simulink model "simple_router"  (R2015a)
settings: Solver=ode45  StartTime=0.0  StopTime=3000  FixedStep=1  RelTol=1e-3
undefined symbols (not defined in the file or in its folder): des, SELECT, T
libraries: simulink x16
(part 5 of 6)

== system simple_router/Router13/Clocked FIFO5 ==
  Event-Based Random Number : EventBasedRandomNumber  Distribution=Gaussian (normal)  meanNorm=E  stdNorm=S
  FIFO Queue : FIFOQueue  Capacity=F  StatNumberInBlock=on
      settings: OutputPortMap=o1
  Release Gate : ReleaseGate  OpenGateUpon=Function call from port fcn
  Time-Based Function-Call Generator : TimeBasedFunctionCallGenerator  EventGenerationMode=Period from port  Period=T
  Input : PMIOPort  Port=1  Side=Left
  Output : PMIOPort  Port=2  Side=Right
  #n : Outport
  wires:
  Time-Based Function-Call Generator/1 -> Release Gate/1
  FIFO Queue/1 -> #n/1
  Event-Based Random Number/1 -> Time-Based Function-Call Generator/1
  connections:
  FIFO Queue/LConn1 -- Input/RConn1
  Release Gate/RConn1 -- Output/RConn1
  FIFO Queue/RConn1 -- Release Gate/LConn1

== system simple_router/Router20/Attribute Function ==
  MATLAB Function : MATLAB Function  TreatAsAtomicUnit=on
  __DMLF__EDE2FCE__ : EntityDepartureFunctionCallGenerator  TimingFunctionCallF1=Before entity departure  IsInsideAFB=on
  __DMLF__GA__ : GetAttribute  AttributeName=DST|ME  AttributeMissing=Error|Error  AttributeDefaultValue=1|1  AttributeTreatAsVector=1|1  AttributeSendTiming=Before entity departure|Before entity departure  EvaluatedDefaultAttributeValue={ [];[]}  IsInsideAFB=on
      settings: OutputPortMap=o1,o2
  __DMLF__SA__ : SetAttribute  AttributeName=RT  AttributeFrom=Signal port  EvaluatedAttributeValue={ []}  IsInsideAFB=on
  IN : PMIOPort  Port=1  Side=Left
  OUT : PMIOPort  Port=2  Side=Right
  wires:
  __DMLF__EDE2FCE__/1 -> MATLAB Function/Trigger
  __DMLF__GA__/1 -> MATLAB Function/1(DST)
  __DMLF__GA__/2 -> MATLAB Function/2(ME)
  MATLAB Function/1(out_RT) -> __DMLF__SA__/1
  connections:
  __DMLF__SA__/LConn1 -- __DMLF__EDE2FCE__/RConn1
  __DMLF__GA__/RConn1 -- __DMLF__EDE2FCE__/LConn1
  IN/RConn1 -- __DMLF__GA__/LConn1
  __DMLF__SA__/RConn1 -- OUT/RConn1

== system simple_router/Router20/Clocked FIFO1 ==
  Event-Based Random Number : EventBasedRandomNumber  Distribution=Gaussian (normal)  meanNorm=E  stdNorm=S
  FIFO Queue : FIFOQueue  Capacity=F  StatNumberInBlock=on
      settings: OutputPortMap=o1
  Release Gate : ReleaseGate  OpenGateUpon=Function call from port fcn
  Time-Based Function-Call Generator : TimeBasedFunctionCallGenerator  EventGenerationMode=Period from port  Period=T
  Input : PMIOPort  Port=1  Side=Left
  Output : PMIOPort  Port=2  Side=Right
  #n : Outport
  wires:
  Time-Based Function-Call Generator/1 -> Release Gate/1
  FIFO Queue/1 -> #n/1
  Event-Based Random Number/1 -> Time-Based Function-Call Generator/1
  connections:
  FIFO Queue/LConn1 -- Input/RConn1
  Release Gate/RConn1 -- Output/RConn1
  FIFO Queue/RConn1 -- Release Gate/LConn1

== system simple_router/Router20/Clocked FIFO2 ==
  Event-Based Random Number : EventBasedRandomNumber  Distribution=Gaussian (normal)  meanNorm=E  stdNorm=S
  FIFO Queue : FIFOQueue  Capacity=F  StatNumberInBlock=on
      settings: OutputPortMap=o1
  Release Gate : ReleaseGate  OpenGateUpon=Function call from port fcn
  Time-Based Function-Call Generator : TimeBasedFunctionCallGenerator  EventGenerationMode=Period from port  Period=T
  Input : PMIOPort  Port=1  Side=Left
  Output : PMIOPort  Port=2  Side=Right
  #n : Outport
  wires:
  Time-Based Function-Call Generator/1 -> Release Gate/1
  FIFO Queue/1 -> #n/1
  Event-Based Random Number/1 -> Time-Based Function-Call Generator/1
  connections:
  FIFO Queue/LConn1 -- Input/RConn1
  Release Gate/RConn1 -- Output/RConn1
  FIFO Queue/RConn1 -- Release Gate/LConn1

== system simple_router/Router20/Clocked FIFO3 ==
  Event-Based Random Number : EventBasedRandomNumber  Distribution=Gaussian (normal)  meanNorm=E  stdNorm=S
  FIFO Queue : FIFOQueue  Capacity=F  StatNumberInBlock=on
      settings: OutputPortMap=o1
  Release Gate : ReleaseGate  OpenGateUpon=Function call from port fcn
  Time-Based Function-Call Generator : TimeBasedFunctionCallGenerator  EventGenerationMode=Period from port  Period=T
  Input : PMIOPort  Port=1  Side=Left
  Output : PMIOPort  Port=2  Side=Right
  #n : Outport
  wires:
  Time-Based Function-Call Generator/1 -> Release Gate/1
  FIFO Queue/1 -> #n/1
  Event-Based Random Number/1 -> Time-Based Function-Call Generator/1
  connections:
  FIFO Queue/LConn1 -- Input/RConn1
  Release Gate/RConn1 -- Output/RConn1
  FIFO Queue/RConn1 -- Release Gate/LConn1

== system simple_router/Router20/Clocked FIFO4 ==
  Event-Based Random Number : EventBasedRandomNumber  Distribution=Gaussian (normal)  meanNorm=E  stdNorm=S
  FIFO Queue : FIFOQueue  Capacity=F  StatNumberInBlock=on
      settings: OutputPortMap=o1
  Release Gate : ReleaseGate  OpenGateUpon=Function call from port fcn
  Time-Based Function-Call Generator : TimeBasedFunctionCallGenerator  EventGenerationMode=Period from port  Period=T
  Input : PMIOPort  Port=1  Side=Left
  Output : PMIOPort  Port=2  Side=Right
  #n : Outport
  wires:
  Time-Based Function-Call Generator/1 -> Release Gate/1
  FIFO Queue/1 -> #n/1
  Event-Based Random Number/1 -> Time-Based Function-Call Generator/1
  connections:
  FIFO Queue/LConn1 -- Input/RConn1
  Release Gate/RConn1 -- Output/RConn1
  FIFO Queue/RConn1 -- Release Gate/LConn1

== system simple_router/Router20/Clocked FIFO5 ==
  Event-Based Random Number : EventBasedRandomNumber  Distribution=Gaussian (normal)  meanNorm=E  stdNorm=S
  FIFO Queue : FIFOQueue  Capacity=F  StatNumberInBlock=on
      settings: OutputPortMap=o1
  Release Gate : ReleaseGate  OpenGateUpon=Function call from port fcn
  Time-Based Function-Call Generator : TimeBasedFunctionCallGenerator  EventGenerationMode=Period from port  Period=T
  Input : PMIOPort  Port=1  Side=Left
  Output : PMIOPort  Port=2  Side=Right
  #n : Outport
  wires:
  Time-Based Function-Call Generator/1 -> Release Gate/1
  FIFO Queue/1 -> #n/1
  Event-Based Random Number/1 -> Time-Based Function-Call Generator/1
  connections:
  FIFO Queue/LConn1 -- Input/RConn1
  Release Gate/RConn1 -- Output/RConn1
  FIFO Queue/RConn1 -- Release Gate/LConn1

== system simple_router/Router22/Attribute Function ==
  MATLAB Function : MATLAB Function  TreatAsAtomicUnit=on
  __DMLF__EDE2FCE__ : EntityDepartureFunctionCallGenerator  TimingFunctionCallF1=Before entity departure  IsInsideAFB=on
  __DMLF__GA__ : GetAttribute  AttributeName=DST|ME  AttributeMissing=Error|Error  AttributeDefaultValue=1|1  AttributeTreatAsVector=1|1  AttributeSendTiming=Before entity departure|Before entity departure  EvaluatedDefaultAttributeValue={ [];[]}  IsInsideAFB=on
      settings: OutputPortMap=o1,o2
  __DMLF__SA__ : SetAttribute  AttributeName=RT  AttributeFrom=Signal port  EvaluatedAttributeValue={ []}  IsInsideAFB=on
  IN : PMIOPort  Port=1  Side=Left
  OUT : PMIOPort  Port=2  Side=Right
  wires:
  __DMLF__EDE2FCE__/1 -> MATLAB Function/Trigger
  __DMLF__GA__/1 -> MATLAB Function/1(DST)
  __DMLF__GA__/2 -> MATLAB Function/2(ME)
  MATLAB Function/1(out_RT) -> __DMLF__SA__/1
  connections:
  __DMLF__SA__/LConn1 -- __DMLF__EDE2FCE__/RConn1
  __DMLF__GA__/RConn1 -- __DMLF__EDE2FCE__/LConn1
  IN/RConn1 -- __DMLF__GA__/LConn1
  __DMLF__SA__/RConn1 -- OUT/RConn1

== system simple_router/Router22/Clocked FIFO1 ==
  Event-Based Random Number : EventBasedRandomNumber  Distribution=Gaussian (normal)  meanNorm=E  stdNorm=S
  FIFO Queue : FIFOQueue  Capacity=F  StatNumberInBlock=on
      settings: OutputPortMap=o1
  Release Gate : ReleaseGate  OpenGateUpon=Function call from port fcn
  Time-Based Function-Call Generator : TimeBasedFunctionCallGenerator  EventGenerationMode=Period from port  Period=T
  Input : PMIOPort  Port=1  Side=Left
  Output : PMIOPort  Port=2  Side=Right
  #n : Outport
  wires:
  Time-Based Function-Call Generator/1 -> Release Gate/1
  FIFO Queue/1 -> #n/1
  Event-Based Random Number/1 -> Time-Based Function-Call Generator/1
  connections:
  FIFO Queue/LConn1 -- Input/RConn1
  Release Gate/RConn1 -- Output/RConn1
  FIFO Queue/RConn1 -- Release Gate/LConn1

== system simple_router/Router22/Clocked FIFO2 ==
  Event-Based Random Number : EventBasedRandomNumber  Distribution=Gaussian (normal)  meanNorm=E  stdNorm=S
  FIFO Queue : FIFOQueue  Capacity=F  StatNumberInBlock=on
      settings: OutputPortMap=o1
  Release Gate : ReleaseGate  OpenGateUpon=Function call from port fcn
  Time-Based Function-Call Generator : TimeBasedFunctionCallGenerator  EventGenerationMode=Period from port  Period=T
  Input : PMIOPort  Port=1  Side=Left
  Output : PMIOPort  Port=2  Side=Right
  #n : Outport
  wires:
  Time-Based Function-Call Generator/1 -> Release Gate/1
  FIFO Queue/1 -> #n/1
  Event-Based Random Number/1 -> Time-Based Function-Call Generator/1
  connections:
  FIFO Queue/LConn1 -- Input/RConn1
  Release Gate/RConn1 -- Output/RConn1
  FIFO Queue/RConn1 -- Release Gate/LConn1

== system simple_router/Router22/Clocked FIFO3 ==
  Event-Based Random Number : EventBasedRandomNumber  Distribution=Gaussian (normal)  meanNorm=E  stdNorm=S
  FIFO Queue : FIFOQueue  Capacity=F  StatNumberInBlock=on
      settings: OutputPortMap=o1
  Release Gate : ReleaseGate  OpenGateUpon=Function call from port fcn
  Time-Based Function-Call Generator : TimeBasedFunctionCallGenerator  EventGenerationMode=Period from port  Period=T
  Input : PMIOPort  Port=1  Side=Left
  Output : PMIOPort  Port=2  Side=Right
  #n : Outport
  wires:
  Time-Based Function-Call Generator/1 -> Release Gate/1
  FIFO Queue/1 -> #n/1
  Event-Based Random Number/1 -> Time-Based Function-Call Generator/1
  connections:
  FIFO Queue/LConn1 -- Input/RConn1
  Release Gate/RConn1 -- Output/RConn1
  FIFO Queue/RConn1 -- Release Gate/LConn1

== system simple_router/Router22/Clocked FIFO4 ==
  Event-Based Random Number : EventBasedRandomNumber  Distribution=Gaussian (normal)  meanNorm=E  stdNorm=S
  FIFO Queue : FIFOQueue  Capacity=F  StatNumberInBlock=on
      settings: OutputPortMap=o1
  Release Gate : ReleaseGate  OpenGateUpon=Function call from port fcn
  Time-Based Function-Call Generator : TimeBasedFunctionCallGenerator  EventGenerationMode=Period from port  Period=T
  Input : PMIOPort  Port=1  Side=Left
  Output : PMIOPort  Port=2  Side=Right
  #n : Outport
  wires:
  Time-Based Function-Call Generator/1 -> Release Gate/1
  FIFO Queue/1 -> #n/1
  Event-Based Random Number/1 -> Time-Based Function-Call Generator/1
  connections:
  FIFO Queue/LConn1 -- Input/RConn1
  Release Gate/RConn1 -- Output/RConn1
  FIFO Queue/RConn1 -- Release Gate/LConn1

== system simple_router/Router22/Clocked FIFO5 ==
  Event-Based Random Number : EventBasedRandomNumber  Distribution=Gaussian (normal)  meanNorm=E  stdNorm=S
  FIFO Queue : FIFOQueue  Capacity=F  StatNumberInBlock=on
      settings: OutputPortMap=o1
  Release Gate : ReleaseGate  OpenGateUpon=Function call from port fcn
  Time-Based Function-Call Generator : TimeBasedFunctionCallGenerator  EventGenerationMode=Period from port  Period=T
  Input : PMIOPort  Port=1  Side=Left
  Output : PMIOPort  Port=2  Side=Right
  #n : Outport
  wires:
  Time-Based Function-Call Generator/1 -> Release Gate/1
  FIFO Queue/1 -> #n/1
  Event-Based Random Number/1 -> Time-Based Function-Call Generator/1
  connections:
  FIFO Queue/LConn1 -- Input/RConn1
  Release Gate/RConn1 -- Output/RConn1
  FIFO Queue/RConn1 -- Release Gate/LConn1

== system simple_router/Router23/Attribute Function ==
  MATLAB Function : MATLAB Function  TreatAsAtomicUnit=on
  __DMLF__EDE2FCE__ : EntityDepartureFunctionCallGenerator  TimingFunctionCallF1=Before entity departure  IsInsideAFB=on
  __DMLF__GA__ : GetAttribute  AttributeName=DST|ME  AttributeMissing=Error|Error  AttributeDefaultValue=1|1  AttributeTreatAsVector=1|1  AttributeSendTiming=Before entity departure|Before entity departure  EvaluatedDefaultAttributeValue={ [];[]}  IsInsideAFB=on
      settings: OutputPortMap=o1,o2
  __DMLF__SA__ : SetAttribute  AttributeName=RT  AttributeFrom=Signal port  EvaluatedAttributeValue={ []}  IsInsideAFB=on
  IN : PMIOPort  Port=1  Side=Left
  OUT : PMIOPort  Port=2  Side=Right
  wires:
  __DMLF__EDE2FCE__/1 -> MATLAB Function/Trigger
  __DMLF__GA__/1 -> MATLAB Function/1(DST)
  __DMLF__GA__/2 -> MATLAB Function/2(ME)
  MATLAB Function/1(out_RT) -> __DMLF__SA__/1
  connections:
  __DMLF__SA__/LConn1 -- __DMLF__EDE2FCE__/RConn1
  __DMLF__GA__/RConn1 -- __DMLF__EDE2FCE__/LConn1
  IN/RConn1 -- __DMLF__GA__/LConn1
  __DMLF__SA__/RConn1 -- OUT/RConn1

== system simple_router/Router23/Clocked FIFO1 ==
  Event-Based Random Number : EventBasedRandomNumber  Distribution=Gaussian (normal)  meanNorm=E  stdNorm=S
  FIFO Queue : FIFOQueue  Capacity=F  StatNumberInBlock=on
      settings: OutputPortMap=o1
  Release Gate : ReleaseGate  OpenGateUpon=Function call from port fcn
  Time-Based Function-Call Generator : TimeBasedFunctionCallGenerator  EventGenerationMode=Period from port  Period=T
  Input : PMIOPort  Port=1  Side=Left
  Output : PMIOPort  Port=2  Side=Right
  #n : Outport
  wires:
  Time-Based Function-Call Generator/1 -> Release Gate/1
  FIFO Queue/1 -> #n/1
  Event-Based Random Number/1 -> Time-Based Function-Call Generator/1
  connections:
  FIFO Queue/LConn1 -- Input/RConn1
  Release Gate/RConn1 -- Output/RConn1
  FIFO Queue/RConn1 -- Release Gate/LConn1

== system simple_router/Router23/Clocked FIFO2 ==
  Event-Based Random Number : EventBasedRandomNumber  Distribution=Gaussian (normal)  meanNorm=E  stdNorm=S
  FIFO Queue : FIFOQueue  Capacity=F  StatNumberInBlock=on
      settings: OutputPortMap=o1
  Release Gate : ReleaseGate  OpenGateUpon=Function call from port fcn
  Time-Based Function-Call Generator : TimeBasedFunctionCallGenerator  EventGenerationMode=Period from port  Period=T
  Input : PMIOPort  Port=1  Side=Left
  Output : PMIOPort  Port=2  Side=Right
  #n : Outport
  wires:
  Time-Based Function-Call Generator/1 -> Release Gate/1
  FIFO Queue/1 -> #n/1
  Event-Based Random Number/1 -> Time-Based Function-Call Generator/1
  connections:
  FIFO Queue/LConn1 -- Input/RConn1
  Release Gate/RConn1 -- Output/RConn1
  FIFO Queue/RConn1 -- Release Gate/LConn1

== system simple_router/Router23/Clocked FIFO3 ==
  Event-Based Random Number : EventBasedRandomNumber  Distribution=Gaussian (normal)  meanNorm=E  stdNorm=S
  FIFO Queue : FIFOQueue  Capacity=F  StatNumberInBlock=on
      settings: OutputPortMap=o1
  Release Gate : ReleaseGate  OpenGateUpon=Function call from port fcn
  Time-Based Function-Call Generator : TimeBasedFunctionCallGenerator  EventGenerationMode=Period from port  Period=T
  Input : PMIOPort  Port=1  Side=Left
  Output : PMIOPort  Port=2  Side=Right
  #n : Outport
  wires:
  Time-Based Function-Call Generator/1 -> Release Gate/1
  FIFO Queue/1 -> #n/1
  Event-Based Random Number/1 -> Time-Based Function-Call Generator/1
  connections:
  FIFO Queue/LConn1 -- Input/RConn1
  Release Gate/RConn1 -- Output/RConn1
  FIFO Queue/RConn1 -- Release Gate/LConn1

== system simple_router/Router23/Clocked FIFO4 ==
  Event-Based Random Number : EventBasedRandomNumber  Distribution=Gaussian (normal)  meanNorm=E  stdNorm=S
  FIFO Queue : FIFOQueue  Capacity=F  StatNumberInBlock=on
      settings: OutputPortMap=o1
  Release Gate : ReleaseGate  OpenGateUpon=Function call from port fcn
  Time-Based Function-Call Generator : TimeBasedFunctionCallGenerator  EventGenerationMode=Period from port  Period=T
  Input : PMIOPort  Port=1  Side=Left
  Output : PMIOPort  Port=2  Side=Right
  #n : Outport
  wires:
  Time-Based Function-Call Generator/1 -> Release Gate/1
  FIFO Queue/1 -> #n/1
  Event-Based Random Number/1 -> Time-Based Function-Call Generator/1
  connections:
  FIFO Queue/LConn1 -- Input/RConn1
  Release Gate/RConn1 -- Output/RConn1
  FIFO Queue/RConn1 -- Release Gate/LConn1

== system simple_router/Router23/Clocked FIFO5 ==
  Event-Based Random Number : EventBasedRandomNumber  Distribution=Gaussian (normal)  meanNorm=E  stdNorm=S
  FIFO Queue : FIFOQueue  Capacity=F  StatNumberInBlock=on
      settings: OutputPortMap=o1
  Release Gate : ReleaseGate  OpenGateUpon=Function call from port fcn
  Time-Based Function-Call Generator : TimeBasedFunctionCallGenerator  EventGenerationMode=Period from port  Period=T
  Input : PMIOPort  Port=1  Side=Left
  Output : PMIOPort  Port=2  Side=Right
  #n : Outport
  wires:
  Time-Based Function-Call Generator/1 -> Release Gate/1
  FIFO Queue/1 -> #n/1
  Event-Based Random Number/1 -> Time-Based Function-Call Generator/1
  connections:
  FIFO Queue/LConn1 -- Input/RConn1
  Release Gate/RConn1 -- Output/RConn1
  FIFO Queue/RConn1 -- Release Gate/LConn1

== system simple_router/Router30/Attribute Function ==
  MATLAB Function : MATLAB Function  TreatAsAtomicUnit=on
  __DMLF__EDE2FCE__ : EntityDepartureFunctionCallGenerator  TimingFunctionCallF1=Before entity departure  IsInsideAFB=on
  __DMLF__GA__ : GetAttribute  AttributeName=DST|ME  AttributeMissing=Error|Error  AttributeDefaultValue=1|1  AttributeTreatAsVector=1|1  AttributeSendTiming=Before entity departure|Before entity departure  EvaluatedDefaultAttributeValue={ [];[]}  IsInsideAFB=on
      settings: OutputPortMap=o1,o2
  __DMLF__SA__ : SetAttribute  AttributeName=RT  AttributeFrom=Signal port  EvaluatedAttributeValue={ []}  IsInsideAFB=on
  IN : PMIOPort  Port=1  Side=Left
  OUT : PMIOPort  Port=2  Side=Right
  wires:
  __DMLF__EDE2FCE__/1 -> MATLAB Function/Trigger
  __DMLF__GA__/1 -> MATLAB Function/1(DST)
  __DMLF__GA__/2 -> MATLAB Function/2(ME)
  MATLAB Function/1(out_RT) -> __DMLF__SA__/1
  connections:
  __DMLF__SA__/LConn1 -- __DMLF__EDE2FCE__/RConn1
  __DMLF__GA__/RConn1 -- __DMLF__EDE2FCE__/LConn1
  IN/RConn1 -- __DMLF__GA__/LConn1
  __DMLF__SA__/RConn1 -- OUT/RConn1

== system simple_router/Router30/Clocked FIFO1 ==
  Event-Based Random Number : EventBasedRandomNumber  Distribution=Gaussian (normal)  meanNorm=E  stdNorm=S
  FIFO Queue : FIFOQueue  Capacity=F  StatNumberInBlock=on
      settings: OutputPortMap=o1
  Release Gate : ReleaseGate  OpenGateUpon=Function call from port fcn
  Time-Based Function-Call Generator : TimeBasedFunctionCallGenerator  EventGenerationMode=Period from port  Period=T
  Input : PMIOPort  Port=1  Side=Left
  Output : PMIOPort  Port=2  Side=Right
  #n : Outport
  wires:
  Time-Based Function-Call Generator/1 -> Release Gate/1
  FIFO Queue/1 -> #n/1
  Event-Based Random Number/1 -> Time-Based Function-Call Generator/1
  connections:
  FIFO Queue/LConn1 -- Input/RConn1
  Release Gate/RConn1 -- Output/RConn1
  FIFO Queue/RConn1 -- Release Gate/LConn1

== system simple_router/Router30/Clocked FIFO2 ==
  Event-Based Random Number : EventBasedRandomNumber  Distribution=Gaussian (normal)  meanNorm=E  stdNorm=S
  FIFO Queue : FIFOQueue  Capacity=F  StatNumberInBlock=on
      settings: OutputPortMap=o1
  Release Gate : ReleaseGate  OpenGateUpon=Function call from port fcn
  Time-Based Function-Call Generator : TimeBasedFunctionCallGenerator  EventGenerationMode=Period from port  Period=T
  Input : PMIOPort  Port=1  Side=Left
  Output : PMIOPort  Port=2  Side=Right
  #n : Outport
  wires:
  Time-Based Function-Call Generator/1 -> Release Gate/1
  FIFO Queue/1 -> #n/1
  Event-Based Random Number/1 -> Time-Based Function-Call Generator/1
  connections:
  FIFO Queue/LConn1 -- Input/RConn1
  Release Gate/RConn1 -- Output/RConn1
  FIFO Queue/RConn1 -- Release Gate/LConn1

== system simple_router/Router30/Clocked FIFO3 ==
  Event-Based Random Number : EventBasedRandomNumber  Distribution=Gaussian (normal)  meanNorm=E  stdNorm=S
  FIFO Queue : FIFOQueue  Capacity=F  StatNumberInBlock=on
      settings: OutputPortMap=o1
  Release Gate : ReleaseGate  OpenGateUpon=Function call from port fcn
  Time-Based Function-Call Generator : TimeBasedFunctionCallGenerator  EventGenerationMode=Period from port  Period=T
  Input : PMIOPort  Port=1  Side=Left
  Output : PMIOPort  Port=2  Side=Right
  #n : Outport
  wires:
  Time-Based Function-Call Generator/1 -> Release Gate/1
  FIFO Queue/1 -> #n/1
  Event-Based Random Number/1 -> Time-Based Function-Call Generator/1
  connections:
  FIFO Queue/LConn1 -- Input/RConn1
  Release Gate/RConn1 -- Output/RConn1
  FIFO Queue/RConn1 -- Release Gate/LConn1

== system simple_router/Router30/Clocked FIFO4 ==
  Event-Based Random Number : EventBasedRandomNumber  Distribution=Gaussian (normal)  meanNorm=E  stdNorm=S
  FIFO Queue : FIFOQueue  Capacity=F  StatNumberInBlock=on
      settings: OutputPortMap=o1
  Release Gate : ReleaseGate  OpenGateUpon=Function call from port fcn
  Time-Based Function-Call Generator : TimeBasedFunctionCallGenerator  EventGenerationMode=Period from port  Period=T
  Input : PMIOPort  Port=1  Side=Left
  Output : PMIOPort  Port=2  Side=Right
  #n : Outport
  wires:
  Time-Based Function-Call Generator/1 -> Release Gate/1
  FIFO Queue/1 -> #n/1
  Event-Based Random Number/1 -> Time-Based Function-Call Generator/1
  connections:
  FIFO Queue/LConn1 -- Input/RConn1
  Release Gate/RConn1 -- Output/RConn1
  FIFO Queue/RConn1 -- Release Gate/LConn1

== system simple_router/Router30/Clocked FIFO5 ==
  Event-Based Random Number : EventBasedRandomNumber  Distribution=Gaussian (normal)  meanNorm=E  stdNorm=S
  FIFO Queue : FIFOQueue  Capacity=F  StatNumberInBlock=on
      settings: OutputPortMap=o1
  Release Gate : ReleaseGate  OpenGateUpon=Function call from port fcn
  Time-Based Function-Call Generator : TimeBasedFunctionCallGenerator  EventGenerationMode=Period from port  Period=T
  Input : PMIOPort  Port=1  Side=Left
  Output : PMIOPort  Port=2  Side=Right
  #n : Outport
  wires:
  Time-Based Function-Call Generator/1 -> Release Gate/1
  FIFO Queue/1 -> #n/1
  Event-Based Random Number/1 -> Time-Based Function-Call Generator/1
  connections:
  FIFO Queue/LConn1 -- Input/RConn1
  Release Gate/RConn1 -- Output/RConn1
  FIFO Queue/RConn1 -- Release Gate/LConn1

== system simple_router/Router31/Attribute Function ==
  MATLAB Function : MATLAB Function  TreatAsAtomicUnit=on
  __DMLF__EDE2FCE__ : EntityDepartureFunctionCallGenerator  TimingFunctionCallF1=Before entity departure  IsInsideAFB=on
  __DMLF__GA__ : GetAttribute  AttributeName=DST|ME  AttributeMissing=Error|Error  AttributeDefaultValue=1|1  AttributeTreatAsVector=1|1  AttributeSendTiming=Before entity departure|Before entity departure  EvaluatedDefaultAttributeValue={ [];[]}  IsInsideAFB=on
      settings: OutputPortMap=o1,o2
  __DMLF__SA__ : SetAttribute  AttributeName=RT  AttributeFrom=Signal port  EvaluatedAttributeValue={ []}  IsInsideAFB=on
  IN : PMIOPort  Port=1  Side=Left
  OUT : PMIOPort  Port=2  Side=Right
  wires:
  __DMLF__EDE2FCE__/1 -> MATLAB Function/Trigger
  __DMLF__GA__/1 -> MATLAB Function/1(DST)
  __DMLF__GA__/2 -> MATLAB Function/2(ME)
  MATLAB Function/1(out_RT) -> __DMLF__SA__/1
  connections:
  __DMLF__SA__/LConn1 -- __DMLF__EDE2FCE__/RConn1
  __DMLF__GA__/RConn1 -- __DMLF__EDE2FCE__/LConn1
  IN/RConn1 -- __DMLF__GA__/LConn1
  __DMLF__SA__/RConn1 -- OUT/RConn1

== system simple_router/Router31/Clocked FIFO1 ==
  Event-Based Random Number : EventBasedRandomNumber  Distribution=Gaussian (normal)  meanNorm=E  stdNorm=S
  FIFO Queue : FIFOQueue  Capacity=F  StatNumberInBlock=on
      settings: OutputPortMap=o1
  Release Gate : ReleaseGate  OpenGateUpon=Function call from port fcn
  Time-Based Function-Call Generator : TimeBasedFunctionCallGenerator  EventGenerationMode=Period from port  Period=T
  Input : PMIOPort  Port=1  Side=Left
  Output : PMIOPort  Port=2  Side=Right
  #n : Outport
  wires:
  Time-Based Function-Call Generator/1 -> Release Gate/1
  FIFO Queue/1 -> #n/1
  Event-Based Random Number/1 -> Time-Based Function-Call Generator/1
  connections:
  FIFO Queue/LConn1 -- Input/RConn1
  Release Gate/RConn1 -- Output/RConn1
  FIFO Queue/RConn1 -- Release Gate/LConn1

== system simple_router/Router31/Clocked FIFO2 ==
  Event-Based Random Number : EventBasedRandomNumber  Distribution=Gaussian (normal)  meanNorm=E  stdNorm=S
  FIFO Queue : FIFOQueue  Capacity=F  StatNumberInBlock=on
      settings: OutputPortMap=o1
  Release Gate : ReleaseGate  OpenGateUpon=Function call from port fcn
  Time-Based Function-Call Generator : TimeBasedFunctionCallGenerator  EventGenerationMode=Period from port  Period=T
  Input : PMIOPort  Port=1  Side=Left
  Output : PMIOPort  Port=2  Side=Right
  #n : Outport
  wires:
  Time-Based Function-Call Generator/1 -> Release Gate/1
  FIFO Queue/1 -> #n/1
  Event-Based Random Number/1 -> Time-Based Function-Call Generator/1
  connections:
  FIFO Queue/LConn1 -- Input/RConn1
  Release Gate/RConn1 -- Output/RConn1
  FIFO Queue/RConn1 -- Release Gate/LConn1

== system simple_router/Router31/Clocked FIFO3 ==
  Event-Based Random Number : EventBasedRandomNumber  Distribution=Gaussian (normal)  meanNorm=E  stdNorm=S
  FIFO Queue : FIFOQueue  Capacity=F  StatNumberInBlock=on
      settings: OutputPortMap=o1
  Release Gate : ReleaseGate  OpenGateUpon=Function call from port fcn
  Time-Based Function-Call Generator : TimeBasedFunctionCallGenerator  EventGenerationMode=Period from port  Period=T
  Input : PMIOPort  Port=1  Side=Left
  Output : PMIOPort  Port=2  Side=Right
  #n : Outport
  wires:
  Time-Based Function-Call Generator/1 -> Release Gate/1
  FIFO Queue/1 -> #n/1
  Event-Based Random Number/1 -> Time-Based Function-Call Generator/1
  connections:
  FIFO Queue/LConn1 -- Input/RConn1
  Release Gate/RConn1 -- Output/RConn1
  FIFO Queue/RConn1 -- Release Gate/LConn1

== system simple_router/Router31/Clocked FIFO4 ==
  Event-Based Random Number : EventBasedRandomNumber  Distribution=Gaussian (normal)  meanNorm=E  stdNorm=S
  FIFO Queue : FIFOQueue  Capacity=F  StatNumberInBlock=on
      settings: OutputPortMap=o1
  Release Gate : ReleaseGate  OpenGateUpon=Function call from port fcn
  Time-Based Function-Call Generator : TimeBasedFunctionCallGenerator  EventGenerationMode=Period from port  Period=T
  Input : PMIOPort  Port=1  Side=Left
  Output : PMIOPort  Port=2  Side=Right
  #n : Outport
  wires:
  Time-Based Function-Call Generator/1 -> Release Gate/1
  FIFO Queue/1 -> #n/1
  Event-Based Random Number/1 -> Time-Based Function-Call Generator/1
  connections:
  FIFO Queue/LConn1 -- Input/RConn1
  Release Gate/RConn1 -- Output/RConn1
  FIFO Queue/RConn1 -- Release Gate/LConn1

== system simple_router/Router31/Clocked FIFO5 ==
  Event-Based Random Number : EventBasedRandomNumber  Distribution=Gaussian (normal)  meanNorm=E  stdNorm=S
  FIFO Queue : FIFOQueue  Capacity=F  StatNumberInBlock=on
      settings: OutputPortMap=o1
  Release Gate : ReleaseGate  OpenGateUpon=Function call from port fcn
  Time-Based Function-Call Generator : TimeBasedFunctionCallGenerator  EventGenerationMode=Period from port  Period=T
  Input : PMIOPort  Port=1  Side=Left
  Output : PMIOPort  Port=2  Side=Right
  #n : Outport
  wires:
  Time-Based Function-Call Generator/1 -> Release Gate/1
  FIFO Queue/1 -> #n/1
  Event-Based Random Number/1 -> Time-Based Function-Call Generator/1
  connections:
  FIFO Queue/LConn1 -- Input/RConn1
  Release Gate/RConn1 -- Output/RConn1
  FIFO Queue/RConn1 -- Release Gate/LConn1

== system simple_router/Router32/Attribute Function ==
  MATLAB Function : MATLAB Function  TreatAsAtomicUnit=on
  __DMLF__EDE2FCE__ : EntityDepartureFunctionCallGenerator  TimingFunctionCallF1=Before entity departure  IsInsideAFB=on
  __DMLF__GA__ : GetAttribute  AttributeName=DST|ME  AttributeMissing=Error|Error  AttributeDefaultValue=1|1  AttributeTreatAsVector=1|1  AttributeSendTiming=Before entity departure|Before entity departure  EvaluatedDefaultAttributeValue={ [];[]}  IsInsideAFB=on
      settings: OutputPortMap=o1,o2
  __DMLF__SA__ : SetAttribute  AttributeName=RT  AttributeFrom=Signal port  EvaluatedAttributeValue={ []}  IsInsideAFB=on
  IN : PMIOPort  Port=1  Side=Left
  OUT : PMIOPort  Port=2  Side=Right
  wires:
  __DMLF__EDE2FCE__/1 -> MATLAB Function/Trigger
  __DMLF__GA__/1 -> MATLAB Function/1(DST)
  __DMLF__GA__/2 -> MATLAB Function/2(ME)
  MATLAB Function/1(out_RT) -> __DMLF__SA__/1
  connections:
  __DMLF__SA__/LConn1 -- __DMLF__EDE2FCE__/RConn1
  __DMLF__GA__/RConn1 -- __DMLF__EDE2FCE__/LConn1
  IN/RConn1 -- __DMLF__GA__/LConn1
  __DMLF__SA__/RConn1 -- OUT/RConn1

== system simple_router/Router32/Clocked FIFO1 ==
  Event-Based Random Number : EventBasedRandomNumber  Distribution=Gaussian (normal)  meanNorm=E  stdNorm=S
  FIFO Queue : FIFOQueue  Capacity=F  StatNumberInBlock=on
      settings: OutputPortMap=o1
  Release Gate : ReleaseGate  OpenGateUpon=Function call from port fcn
  Time-Based Function-Call Generator : TimeBasedFunctionCallGenerator  EventGenerationMode=Period from port  Period=T
  Input : PMIOPort  Port=1  Side=Left
  Output : PMIOPort  Port=2  Side=Right
  #n : Outport
  wires:
  Time-Based Function-Call Generator/1 -> Release Gate/1
  FIFO Queue/1 -> #n/1
  Event-Based Random Number/1 -> Time-Based Function-Call Generator/1
  connections:
  FIFO Queue/LConn1 -- Input/RConn1
  Release Gate/RConn1 -- Output/RConn1
  FIFO Queue/RConn1 -- Release Gate/LConn1

== system simple_router/Router32/Clocked FIFO2 ==
  Event-Based Random Number : EventBasedRandomNumber  Distribution=Gaussian (normal)  meanNorm=E  stdNorm=S
  FIFO Queue : FIFOQueue  Capacity=F  StatNumberInBlock=on
      settings: OutputPortMap=o1
  Release Gate : ReleaseGate  OpenGateUpon=Function call from port fcn
  Time-Based Function-Call Generator : TimeBasedFunctionCallGenerator  EventGenerationMode=Period from port  Period=T
  Input : PMIOPort  Port=1  Side=Left
  Output : PMIOPort  Port=2  Side=Right
  #n : Outport
  wires:
  Time-Based Function-Call Generator/1 -> Release Gate/1
  FIFO Queue/1 -> #n/1
  Event-Based Random Number/1 -> Time-Based Function-Call Generator/1
  connections:
  FIFO Queue/LConn1 -- Input/RConn1
  Release Gate/RConn1 -- Output/RConn1
  FIFO Queue/RConn1 -- Release Gate/LConn1

== system simple_router/Router32/Clocked FIFO3 ==
  Event-Based Random Number : EventBasedRandomNumber  Distribution=Gaussian (normal)  meanNorm=E  stdNorm=S
  FIFO Queue : FIFOQueue  Capacity=F  StatNumberInBlock=on
      settings: OutputPortMap=o1
  Release Gate : ReleaseGate  OpenGateUpon=Function call from port fcn
  Time-Based Function-Call Generator : TimeBasedFunctionCallGenerator  EventGenerationMode=Period from port  Period=T
  Input : PMIOPort  Port=1  Side=Left
  Output : PMIOPort  Port=2  Side=Right
  #n : Outport
  wires:
  Time-Based Function-Call Generator/1 -> Release Gate/1
  FIFO Queue/1 -> #n/1
  Event-Based Random Number/1 -> Time-Based Function-Call Generator/1
  connections:
  FIFO Queue/LConn1 -- Input/RConn1
  Release Gate/RConn1 -- Output/RConn1
  FIFO Queue/RConn1 -- Release Gate/LConn1

== system simple_router/Router32/Clocked FIFO4 ==
  Event-Based Random Number : EventBasedRandomNumber  Distribution=Gaussian (normal)  meanNorm=E  stdNorm=S
  FIFO Queue : FIFOQueue  Capacity=F  StatNumberInBlock=on
      settings: OutputPortMap=o1
  Release Gate : ReleaseGate  OpenGateUpon=Function call from port fcn
  Time-Based Function-Call Generator : TimeBasedFunctionCallGenerator  EventGenerationMode=Period from port  Period=T
  Input : PMIOPort  Port=1  Side=Left
  Output : PMIOPort  Port=2  Side=Right
  #n : Outport
  wires:
  Time-Based Function-Call Generator/1 -> Release Gate/1
  FIFO Queue/1 -> #n/1
  Event-Based Random Number/1 -> Time-Based Function-Call Generator/1
  connections:
  FIFO Queue/LConn1 -- Input/RConn1
  Release Gate/RConn1 -- Output/RConn1
  FIFO Queue/RConn1 -- Release Gate/LConn1

== system simple_router/Router32/Clocked FIFO5 ==
  Event-Based Random Number : EventBasedRandomNumber  Distribution=Gaussian (normal)  meanNorm=E  stdNorm=S
  FIFO Queue : FIFOQueue  Capacity=F  StatNumberInBlock=on
      settings: OutputPortMap=o1
  Release Gate : ReleaseGate  OpenGateUpon=Function call from port fcn
  Time-Based Function-Call Generator : TimeBasedFunctionCallGenerator  EventGenerationMode=Period from port  Period=T
  Input : PMIOPort  Port=1  Side=Left
  Output : PMIOPort  Port=2  Side=Right
  #n : Outport
  wires:
  Time-Based Function-Call Generator/1 -> Release Gate/1
  FIFO Queue/1 -> #n/1
  Event-Based Random Number/1 -> Time-Based Function-Call Generator/1
  connections:
  FIFO Queue/LConn1 -- Input/RConn1
  Release Gate/RConn1 -- Output/RConn1
  FIFO Queue/RConn1 -- Release Gate/LConn1

== system simple_router/Router33/Attribute Function ==
  MATLAB Function : MATLAB Function  TreatAsAtomicUnit=on
  __DMLF__EDE2FCE__ : EntityDepartureFunctionCallGenerator  TimingFunctionCallF1=Before entity departure  IsInsideAFB=on
  __DMLF__GA__ : GetAttribute  AttributeName=DST|ME  AttributeMissing=Error|Error  AttributeDefaultValue=1|1  AttributeTreatAsVector=1|1  AttributeSendTiming=Before entity departure|Before entity departure  EvaluatedDefaultAttributeValue={ [];[]}  IsInsideAFB=on
      settings: OutputPortMap=o1,o2
  __DMLF__SA__ : SetAttribute  AttributeName=RT  AttributeFrom=Signal port  EvaluatedAttributeValue={ []}  IsInsideAFB=on
  IN : PMIOPort  Port=1  Side=Left
  OUT : PMIOPort  Port=2  Side=Right
  wires:
  __DMLF__EDE2FCE__/1 -> MATLAB Function/Trigger
  __DMLF__GA__/1 -> MATLAB Function/1(DST)
  __DMLF__GA__/2 -> MATLAB Function/2(ME)
  MATLAB Function/1(out_RT) -> __DMLF__SA__/1
  connections:
  __DMLF__SA__/LConn1 -- __DMLF__EDE2FCE__/RConn1
  __DMLF__GA__/RConn1 -- __DMLF__EDE2FCE__/LConn1
  IN/RConn1 -- __DMLF__GA__/LConn1
  __DMLF__SA__/RConn1 -- OUT/RConn1

== system simple_router/Router33/Clocked FIFO1 ==
  Event-Based Random Number : EventBasedRandomNumber  Distribution=Gaussian (normal)  meanNorm=E  stdNorm=S
  FIFO Queue : FIFOQueue  Capacity=F  StatNumberInBlock=on
      settings: OutputPortMap=o1
  Release Gate : ReleaseGate  OpenGateUpon=Function call from port fcn
  Time-Based Function-Call Generator : TimeBasedFunctionCallGenerator  EventGenerationMode=Period from port  Period=T
  Input : PMIOPort  Port=1  Side=Left
  Output : PMIOPort  Port=2  Side=Right
  #n : Outport
  wires:
  Time-Based Function-Call Generator/1 -> Release Gate/1
  FIFO Queue/1 -> #n/1
  Event-Based Random Number/1 -> Time-Based Function-Call Generator/1
  connections:
  FIFO Queue/LConn1 -- Input/RConn1
  Release Gate/RConn1 -- Output/RConn1
  FIFO Queue/RConn1 -- Release Gate/LConn1

== system simple_router/Router33/Clocked FIFO2 ==
  Event-Based Random Number : EventBasedRandomNumber  Distribution=Gaussian (normal)  meanNorm=E  stdNorm=S
  FIFO Queue : FIFOQueue  Capacity=F  StatNumberInBlock=on
      settings: OutputPortMap=o1
  Release Gate : ReleaseGate  OpenGateUpon=Function call from port fcn
  Time-Based Function-Call Generator : TimeBasedFunctionCallGenerator  EventGenerationMode=Period from port  Period=T
  Input : PMIOPort  Port=1  Side=Left
  Output : PMIOPort  Port=2  Side=Right
  #n : Outport
  wires:
  Time-Based Function-Call Generator/1 -> Release Gate/1
  FIFO Queue/1 -> #n/1
  Event-Based Random Number/1 -> Time-Based Function-Call Generator/1
  connections:
  FIFO Queue/LConn1 -- Input/RConn1
  Release Gate/RConn1 -- Output/RConn1
  FIFO Queue/RConn1 -- Release Gate/LConn1

== system simple_router/Router33/Clocked FIFO3 ==
  Event-Based Random Number : EventBasedRandomNumber  Distribution=Gaussian (normal)  meanNorm=E  stdNorm=S
  FIFO Queue : FIFOQueue  Capacity=F  StatNumberInBlock=on
      settings: OutputPortMap=o1
  Release Gate : ReleaseGate  OpenGateUpon=Function call from port fcn
  Time-Based Function-Call Generator : TimeBasedFunctionCallGenerator  EventGenerationMode=Period from port  Period=T
  Input : PMIOPort  Port=1  Side=Left
  Output : PMIOPort  Port=2  Side=Right
  #n : Outport
  wires:
  Time-Based Function-Call Generator/1 -> Release Gate/1
  FIFO Queue/1 -> #n/1
  Event-Based Random Number/1 -> Time-Based Function-Call Generator/1
  connections:
  FIFO Queue/LConn1 -- Input/RConn1
  Release Gate/RConn1 -- Output/RConn1
  FIFO Queue/RConn1 -- Release Gate/LConn1

== system simple_router/Router33/Clocked FIFO4 ==
  Event-Based Random Number : EventBasedRandomNumber  Distribution=Gaussian (normal)  meanNorm=E  stdNorm=S
  FIFO Queue : FIFOQueue  Capacity=F  StatNumberInBlock=on
      settings: OutputPortMap=o1
  Release Gate : ReleaseGate  OpenGateUpon=Function call from port fcn
  Time-Based Function-Call Generator : TimeBasedFunctionCallGenerator  EventGenerationMode=Period from port  Period=T
  Input : PMIOPort  Port=1  Side=Left
  Output : PMIOPort  Port=2  Side=Right
  #n : Outport
  wires:
  Time-Based Function-Call Generator/1 -> Release Gate/1
  FIFO Queue/1 -> #n/1
  Event-Based Random Number/1 -> Time-Based Function-Call Generator/1
  connections:
  FIFO Queue/LConn1 -- Input/RConn1
  Release Gate/RConn1 -- Output/RConn1
  FIFO Queue/RConn1 -- Release Gate/LConn1

== system simple_router/Router33/Clocked FIFO5 ==
  Event-Based Random Number : EventBasedRandomNumber  Distribution=Gaussian (normal)  meanNorm=E  stdNorm=S
  FIFO Queue : FIFOQueue  Capacity=F  StatNumberInBlock=on
      settings: OutputPortMap=o1
  Release Gate : ReleaseGate  OpenGateUpon=Function call from port fcn
  Time-Based Function-Call Generator : TimeBasedFunctionCallGenerator  EventGenerationMode=Period from port  Period=T
  Input : PMIOPort  Port=1  Side=Left
  Output : PMIOPort  Port=2  Side=Right
  #n : Outport
  wires:
  Time-Based Function-Call Generator/1 -> Release Gate/1
  FIFO Queue/1 -> #n/1
  Event-Based Random Number/1 -> Time-Based Function-Call Generator/1
  connections:
  FIFO Queue/LConn1 -- Input/RConn1
  Release Gate/RConn1 -- Output/RConn1
  FIFO Queue/RConn1 -- Release Gate/LConn1

== matlab function simple_router/Router00/Attribute Function/MATLAB Function ==
  data: DST input; out_RT output; ME input
  events: trigger input FUNCTION_CALL_EVENT
function out_RT  = fcn(DST,ME)
%FCN    Access and modify attributes with MATLAB 
% 
% Input arguments must match the attribute names.
% Output arguments must be out_<AttributeName>,
% e.g., out_ServiceTime where ServiceTime is the attribute name.
% 
% The output attribute will be created if it is not present.
%

yi = floor(ME/4)+1;
xi = mod(ME,4);

if (xi==0),
    xi = 4;
    yi = yi - 1;
end

y = floor(DST/4)+1;
x = mod(DST,4);

if (x==0),
   x = 4;
    y = y - 1;
end

if x~=xi,
    if (x<xi),
        out_RT = 2;
    else 
        out_RT = 3;
    end
elseif y~=yi,
    if (y<yi),
        out_RT = 1;
    else
        out_RT = 4;
    end
else
    out_RT = 5;
end

== matlab function simple_router/Router01/Attribute Function/MATLAB Function ==
  data: DST input; out_RT output; ME input
  events: trigger input FUNCTION_CALL_EVENT
function out_RT  = fcn(DST,ME)
%FCN    Access and modify attributes with MATLAB 
% 
% Input arguments must match the attribute names.
% Output arguments must be out_<AttributeName>,
% e.g., out_ServiceTime where ServiceTime is the attribute name.
% 
% The output attribute will be created if it is not present.
%

yi = floor(ME/4)+1;
xi = mod(ME,4);

if (xi==0),
    xi = 4;
    yi = yi - 1;
end

y = floor(DST/4)+1;
x = mod(DST,4);

if (x==0),
   x = 4;
    y = y - 1;
end

if x~=xi,
    if (x<xi),
        out_RT = 2;
    else 
        out_RT = 3;
    end
elseif y~=yi,
    if (y<yi),
        out_RT = 1;
    else
        out_RT = 4;
    end
else
    out_RT = 5;
end

== matlab function simple_router/Router02/Attribute Function/MATLAB Function ==
  data: DST input; out_RT output; ME input
  events: trigger input FUNCTION_CALL_EVENT
function out_RT  = fcn(DST,ME)
%FCN    Access and modify attributes with MATLAB 
% 
% Input arguments must match the attribute names.
% Output arguments must be out_<AttributeName>,
% e.g., out_ServiceTime where ServiceTime is the attribute name.
% 
% The output attribute will be created if it is not present.
%

yi = floor(ME/4)+1;
xi = mod(ME,4);

if (xi==0),
    xi = 4;
    yi = yi - 1;
end

y = floor(DST/4)+1;
x = mod(DST,4);

if (x==0),
   x = 4;
    y = y - 1;
end

if x~=xi,
    if (x<xi),
        out_RT = 2;
    else 
        out_RT = 3;
    end
elseif y~=yi,
    if (y<yi),
        out_RT = 1;
    else
        out_RT = 4;
    end
else
    out_RT = 5;
end

== matlab function simple_router/Router03/Attribute Function/MATLAB Function ==
  data: DST input; out_RT output; ME input
  events: trigger input FUNCTION_CALL_EVENT
function out_RT  = fcn(DST,ME)
%FCN    Access and modify attributes with MATLAB 
% 
% Input arguments must match the attribute names.
% Output arguments must be out_<AttributeName>,
% e.g., out_ServiceTime where ServiceTime is the attribute name.
% 
% The output attribute will be created if it is not present.
%

yi = floor(ME/4)+1;
xi = mod(ME,4);

if (xi==0),
    xi = 4;
    yi = yi - 1;
end

y = floor(DST/4)+1;
x = mod(DST,4);

if (x==0),
   x = 4;
    y = y - 1;
end

if x~=xi,
    if (x<xi),
        out_RT = 2;
    else 
        out_RT = 3;
    end
elseif y~=yi,
    if (y<yi),
        out_RT = 1;
    else
        out_RT = 4;
    end
else
    out_RT = 5;
end

== matlab function simple_router/Router10/Attribute Function/MATLAB Function ==
  data: DST input; out_RT output; ME input
  events: trigger input FUNCTION_CALL_EVENT
function out_RT  = fcn(DST,ME)
%FCN    Access and modify attributes with MATLAB 
% 
% Input arguments must match the attribute names.
% Output arguments must be out_<AttributeName>,
% e.g., out_ServiceTime where ServiceTime is the attribute name.
% 
% The output attribute will be created if it is not present.
%

yi = floor(ME/4)+1;
xi = mod(ME,4);

if (xi==0),
    xi = 4;
    yi = yi - 1;
end

y = floor(DST/4)+1;
x = mod(DST,4);

if (x==0),
   x = 4;
    y = y - 1;
end

if x~=xi,
    if (x<xi),
        out_RT = 2;
    else 
        out_RT = 3;
    end
elseif y~=yi,
    if (y<yi),
        out_RT = 1;
    else
        out_RT = 4;
    end
else
    out_RT = 5;
end

== matlab function simple_router/Router11/Attribute Function/MATLAB Function ==
  data: DST input; out_RT output; ME input
  events: trigger input FUNCTION_CALL_EVENT
function out_RT  = fcn(DST,ME)
%FCN    Access and modify attributes with MATLAB 
% 
% Input arguments must match the attribute names.
% Output arguments must be out_<AttributeName>,
% e.g., out_ServiceTime where ServiceTime is the attribute name.
% 
% The output attribute will be created if it is not present.
%

yi = floor(ME/4)+1;
xi = mod(ME,4);

if (xi==0),
    xi = 4;
    yi = yi - 1;
end

y = floor(DST/4)+1;
x = mod(DST,4);

if (x==0),
   x = 4;
    y = y - 1;
end

if x~=xi,
    if (x<xi),
        out_RT = 2;
    else 
        out_RT = 3;
    end
elseif y~=yi,
    if (y<yi),
        out_RT = 1;
    else
        out_RT = 4;
    end
else
    out_RT = 5;
end

== matlab function simple_router/Router12/Attribute Function/MATLAB Function ==
  data: DST input; out_RT output; ME input
  events: trigger input FUNCTION_CALL_EVENT
function out_RT  = fcn(DST,ME)
%FCN    Access and modify attributes with MATLAB 
% 
% Input arguments must match the attribute names.
% Output arguments must be out_<AttributeName>,
% e.g., out_ServiceTime where ServiceTime is the attribute name.
% 
% The output attribute will be created if it is not present.
%

yi = floor(ME/4)+1;
xi = mod(ME,4);

if (xi==0),
    xi = 4;
    yi = yi - 1;
end

y = floor(DST/4)+1;
x = mod(DST,4);

if (x==0),
   x = 4;
    y = y - 1;
end

if x~=xi,
    if (x<xi),
        out_RT = 2;
    else 
        out_RT = 3;
    end
elseif y~=yi,
    if (y<yi),
        out_RT = 1;
    else
        out_RT = 4;
    end
else
    out_RT = 5;
end

== matlab function simple_router/Router13/Attribute Function/MATLAB Function ==
  data: DST input; out_RT output; ME input
  events: trigger input FUNCTION_CALL_EVENT
function out_RT  = fcn(DST,ME)
%FCN    Access and modify attributes with MATLAB 
% 
% Input arguments must match the attribute names.
% Output arguments must be out_<AttributeName>,
% e.g., out_ServiceTime where ServiceTime is the attribute name.
% 
% The output attribute will be created if it is not present.
%

yi = floor(ME/4)+1;
xi = mod(ME,4);

if (xi==0),
    xi = 4;
    yi = yi - 1;
end

y = floor(DST/4)+1;
x = mod(DST,4);

if (x==0),
   x = 4;
    y = y - 1;
end

if x~=xi,
    if (x<xi),
        out_RT = 2;
    else 
        out_RT = 3;
    end
elseif y~=yi,
    if (y<yi),
        out_RT = 1;
    else
        out_RT = 4;
    end
else
    out_RT = 5;
end

== matlab function simple_router/Router22/Attribute Function/MATLAB Function ==
  data: DST input; out_RT output; ME input
  events: trigger input FUNCTION_CALL_EVENT
function out_RT  = fcn(DST,ME)
%FCN    Access and modify attributes with MATLAB 
% 
% Input arguments must match the attribute names.
% Output arguments must be out_<AttributeName>,
% e.g., out_ServiceTime where ServiceTime is the attribute name.
% 
% The output attribute will be created if it is not present.
%

yi = floor(ME/4)+1;
xi = mod(ME,4);

if (xi==0),
    xi = 4;
    yi = yi - 1;
end

y = floor(DST/4)+1;
x = mod(DST,4);

if (x==0),
   x = 4;
    y = y - 1;
end

if x~=xi,
    if (x<xi),
        out_RT = 2;
    else 
        out_RT = 3;
    end
elseif y~=yi,
    if (y<yi),
        out_RT = 1;
    else
        out_RT = 4;
    end
else
    out_RT = 5;
end

== matlab function simple_router/Router23/Attribute Function/MATLAB Function ==
  data: DST input; out_RT output; ME input
  events: trigger input FUNCTION_CALL_EVENT
function out_RT  = fcn(DST,ME)
%FCN    Access and modify attributes with MATLAB 
% 
% Input arguments must match the attribute names.
% Output arguments must be out_<AttributeName>,
% e.g., out_ServiceTime where ServiceTime is the attribute name.
% 
% The output attribute will be created if it is not present.
%

yi = floor(ME/4)+1;
xi = mod(ME,4);

if (xi==0),
    xi = 4;
    yi = yi - 1;
end

y = floor(DST/4)+1;
x = mod(DST,4);

if (x==0),
   x = 4;
    y = y - 1;
end

if x~=xi,
    if (x<xi),
        out_RT = 2;
    else 
        out_RT = 3;
    end
elseif y~=yi,
    if (y<yi),
        out_RT = 1;
    else
        out_RT = 4;
    end
else
    out_RT = 5;
end

== matlab function simple_router/Router20/Attribute Function/MATLAB Function ==
  data: DST input; out_RT output; ME input
  events: trigger input FUNCTION_CALL_EVENT
function out_RT  = fcn(DST,ME)
%FCN    Access and modify attributes with MATLAB 
% 
% Input arguments must match the attribute names.
% Output arguments must be out_<AttributeName>,
% e.g., out_ServiceTime where ServiceTime is the attribute name.
% 
% The output attribute will be created if it is not present.
%

yi = floor(ME/4)+1;
xi = mod(ME,4);

if (xi==0),
    xi = 4;
    yi = yi - 1;
end

y = floor(DST/4)+1;
x = mod(DST,4);

if (x==0),
   x = 4;
    y = y - 1;
end

if x~=xi,
    if (x<xi),
        out_RT = 2;
    else 
        out_RT = 3;
    end
elseif y~=yi,
    if (y<yi),
        out_RT = 1;
    else
        out_RT = 4;
    end
else
    out_RT = 5;
end

== matlab function simple_router/Router09/Attribute Function/MATLAB Function ==
  data: DST input; out_RT output; ME input
  events: trigger input FUNCTION_CALL_EVENT
function out_RT  = fcn(DST,ME)
%FCN    Access and modify attributes with MATLAB 
% 
% Input arguments must match the attribute names.
% Output arguments must be out_<AttributeName>,
% e.g., out_ServiceTime where ServiceTime is the attribute name.
% 
% The output attribute will be created if it is not present.
%

yi = floor(ME/4)+1;
xi = mod(ME,4);

if (xi==0),
    xi = 4;
    yi = yi - 1;
end

y = floor(DST/4)+1;
x = mod(DST,4);

if (x==0),
   x = 4;
    y = y - 1;
end

if x~=xi,
    if (x<xi),
        out_RT = 2;
    else 
        out_RT = 3;
    end
elseif y~=yi,
    if (y<yi),
        out_RT = 1;
    else
        out_RT = 4;
    end
else
    out_RT = 5;
end

== matlab function simple_router/Router30/Attribute Function/MATLAB Function ==
  data: DST input; out_RT output; ME input
  events: trigger input FUNCTION_CALL_EVENT
function out_RT  = fcn(DST,ME)
%FCN    Access and modify attributes with MATLAB 
% 
% Input arguments must match the attribute names.
% Output arguments must be out_<AttributeName>,
% e.g., out_ServiceTime where ServiceTime is the attribute name.
% 
% The output attribute will be created if it is not present.
%

yi = floor(ME/4)+1;
xi = mod(ME,4);

if (xi==0),
    xi = 4;
    yi = yi - 1;
end

y = floor(DST/4)+1;
x = mod(DST,4);

if (x==0),
   x = 4;
    y = y - 1;
end

if x~=xi,
    if (x<xi),
        out_RT = 2;
    else 
        out_RT = 3;
    end
elseif y~=yi,
    if (y<yi),
        out_RT = 1;
    else
        out_RT = 4;
    end
else
    out_RT = 5;
end

== matlab function simple_router/Router31/Attribute Function/MATLAB Function ==
  data: DST input; out_RT output; ME input
  events: trigger input FUNCTION_CALL_EVENT
function out_RT  = fcn(DST,ME)
%FCN    Access and modify attributes with MATLAB 
% 
% Input arguments must match the attribute names.
% Output arguments must be out_<AttributeName>,
% e.g., out_ServiceTime where ServiceTime is the attribute name.
% 
% The output attribute will be created if it is not present.
%

yi = floor(ME/4)+1;
xi = mod(ME,4);

if (xi==0),
    xi = 4;
    yi = yi - 1;
end

y = floor(DST/4)+1;
x = mod(DST,4);

if (x==0),
   x = 4;
    y = y - 1;
end

if x~=xi,
    if (x<xi),
        out_RT = 2;
    else 
        out_RT = 3;
    end
elseif y~=yi,
    if (y<yi),
        out_RT = 1;
    else
        out_RT = 4;
    end
else
    out_RT = 5;
end
